simulink model "SimModel3"  (R2015b)
settings: Solver=VariableStepAuto  StartTime=0.0  StopTime=10.0  RelTol=1e-3
values from neighbouring files (symbols this model uses):
  C1 = [ 1 0]    [Exercise1.m]
  C2 = [0 1]    [Exercise1.m]
  d = 0.5    [Exercise1.m]
  Freq = 10    [Exercise1.m]
  m = 0.1    [Exercise1.m]
  Sine_wave = 1    [Exercise1.m]
undefined symbols (not defined in the file or in its folder): A1, A2, B1, B2, D1, D2, G1den, G1num, G2den, G2num, k
libraries: simulink x1
settings Model: Creator=ooman  LastModifiedBy=sofianh

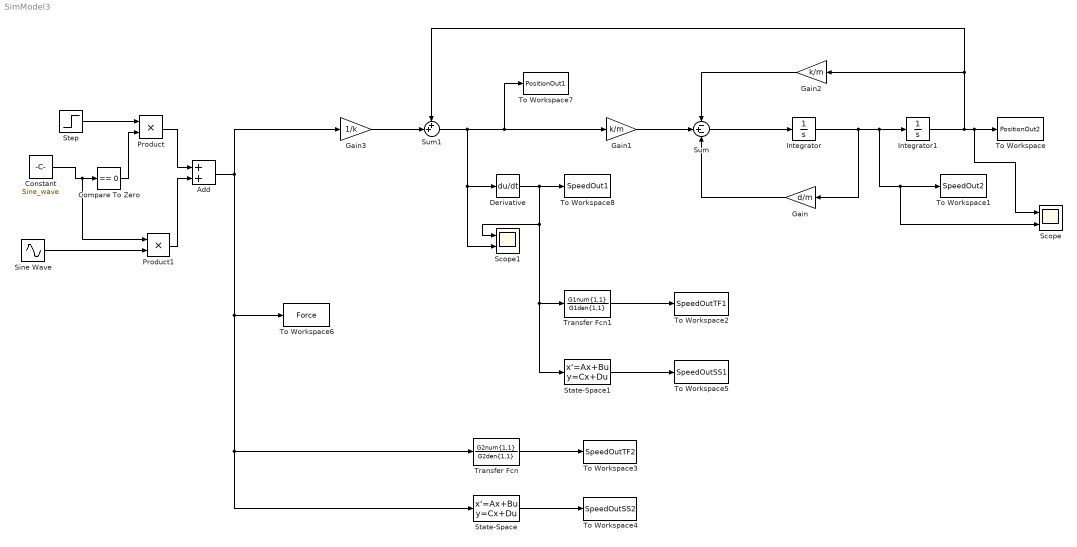
== system SimModel3 ==
  Add : Sum
  Compare To Zero : simulink/Logic and Bit Operations/Compare To Zero  relop===  OutDataTypeStr=boolean
  Constant : Constant  Value=Sine_wave
  Derivative : Derivative
  Gain : Gain  Gain=d/m
  Gain1 : Gain  Gain=k/m
  Gain2 : Gain  Gain=k/m
  Gain3 : Gain  Gain=1/k
  Integrator : Integrator
  Integrator1 : Integrator
  Product : Product
  Product1 : Product
  Scope : Scope  NumInputPorts=2
  Scope1 : Scope  NumInputPorts=2
  Sine Wave : Sin  Frequency=Freq  SampleTime=0
  State-Space : StateSpace  A=A2  B=B2  C=C2  D=D2  X0=0  ContinuousStateAttributes='Speed2'
  State-Space1 : StateSpace  A=A1  B=B1  C=C1  D=D1  X0=0  ContinuousStateAttributes='Speed2'
  Step : Step  Time=0  SampleTime=0
  Sum : Sum  Inputs=-+-
  Sum1 : Sum  Inputs=++|
  To Workspace : ToWorkspace  VariableName=PositionOut2  SaveFormat=Structure With Time  SampleTime=-1
  To Workspace1 : ToWorkspace  VariableName=SpeedOut2  SaveFormat=Structure With Time  SampleTime=-1
  To Workspace2 : ToWorkspace  VariableName=SpeedOutTF1  SaveFormat=Structure With Time  SampleTime=-1
  To Workspace3 : ToWorkspace  VariableName=SpeedOutTF2  SaveFormat=Structure With Time  SampleTime=-1
  To Workspace4 : ToWorkspace  VariableName=SpeedOutSS2  SaveFormat=Structure With Time  SampleTime=-1
  To Workspace5 : ToWorkspace  VariableName=SpeedOutSS1  SaveFormat=Structure With Time  SampleTime=-1
  To Workspace6 : ToWorkspace  VariableName=Force  SaveFormat=Structure With Time  SampleTime=-1
  To Workspace7 : ToWorkspace  VariableName=PositionOut1  SaveFormat=Structure With Time  SampleTime=-1
  To Workspace8 : ToWorkspace  VariableName=SpeedOut1  SaveFormat=Structure With Time  SampleTime=-1
  Transfer Fcn : TransferFcn  Numerator=G2num{1,1}  Denominator=G2den{1,1}  ContinuousStateAttributes='Speed2'
  Transfer Fcn1 : TransferFcn  Numerator=G1num{1,1}  Denominator=G1den{1,1}  ContinuousStateAttributes='Speed2'
  wires:
  Integrator/1 -> Gain/1, Scope/2, To Workspace1/1, Integrator1/1
  Sum/1 -> Integrator/1
  Integrator1/1 -> Gain2/1, Sum1/1, Scope/1, To Workspace/1
  Transfer Fcn/1 -> To Workspace3/1
  State-Space/1 -> To Workspace4/1
  Step/1 -> Product/1
  Constant/1 -> Product1/1, Compare To Zero/1
  Sine Wave/1 -> Product1/2
  Product/1 -> Add/1
  Product1/1 -> Add/2
  Add/1 -> Gain3/1, State-Space/1, Transfer Fcn/1, To Workspace6/1
  Compare To Zero/1 -> Product/2
  Gain1/1 -> Sum/2
  Gain2/1 -> Sum/1
  Gain/1 -> Sum/3
  Gain3/1 -> Sum1/2
  Sum1/1 -> Scope1/2, Derivative/1, To Workspace7/1, Gain1/1
  Transfer Fcn1/1 -> To Workspace2/1
  State-Space1/1 -> To Workspace5/1
  Derivative/1 -> State-Space1/1, Transfer Fcn1/1, Scope1/1, To Workspace8/1
